simulink model "Our_PID_Plain"  (Simulink 8.9)
settings: Solver=VariableStepAuto  StartTime=0.0  StopTime=3000  RelTol=1e-3
settings Model: Creator=maurice waked  LastModifiedBy=maurice waked
settings DataIOCC: LimitDataPoints=off  SaveFormat=Dataset  SignalLoggingSaveFormat=Dataset  ReturnWorkspaceOutputs=on
settings OptimizationCC: LifeSpan=auto
settings DebuggingCC: UnderspecifiedInitializationDetection=Simplified  MergeDetectMultiDrivingBlocksExec=error  FcnCallInpInsideContextMsg=error  StateNameClashWarn=none  SFUnexpectedBacktrackingDiag=error  SFNoUnconditionalDefaultTransitionDiag=error  SFExecutionAtInitializationDiag=warning
settings HardwareCC: ProdBitPerPointer=64  ProdBitPerSizeT=64  ProdBitPerPtrDiffT=64  ProdLargestAtomicFloat=Float  ProdIntDivRoundTo=Zero  ProdEndianess=LittleEndian  ProdWordSize=64  ProdHWDeviceType=Intel->x86-64 (Windows64)
settings ModelReferenceCC: PropagateSignalLabelsOutOfModel=on
settings SFSimCC: SimUseLocalCustomCode=on
settings RTWCC: RTWUseLocalCustomCode=on
settings GRTTargetCC: TargetLangStandard=C99 (ISO)  CombineOutputUpdateFcns=on  GRTInterface=off
settings ConfigComp: CovMetricSettings=dwe  CovHtmlReporting=off  CovSaveCumulativeToWorkspaceVar=off  CovSaveSingleToWorkspaceVar=off  CovExternalEMLEnable=on

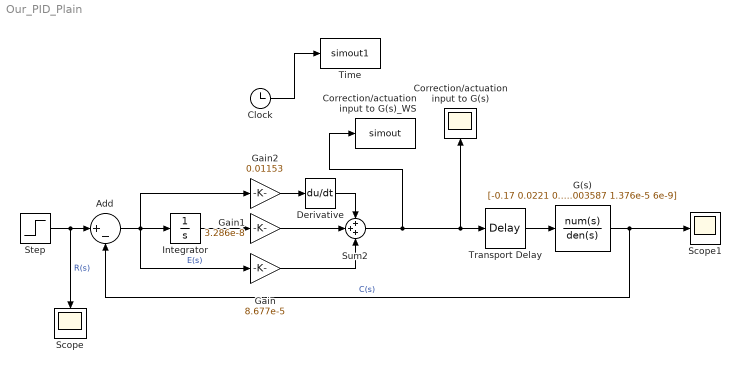
== system Our_PID_Plain ==
  Add : Sum  Inputs=|+-
  Clock : Clock
  Correction/actuation input to G(s) : Scope
  Correction/actuation input to G(s)_WS : ToWorkspace  VariableName=simout  SampleTime=-1
  Derivative : Derivative
  G(s) : TransferFcn  Numerator=[-0.17 0.0221 0.00068]  Denominator=[1 0.1345 0.003587 1.376e-5 6e-9]
  Gain : Gain  Gain=8.677e-5
  Gain1 : Gain  Gain=3.286e-8
  Gain2 : Gain  Gain=0.01153
  Integrator : Integrator
  Scope : Scope
  Scope1 : Scope
  Step : Step  Time=0  SampleTime=0
  Sum2 : Sum  Inputs=+++
  Time : ToWorkspace  VariableName=simout1  SampleTime=-1
  Transport Delay : TransportDelay  DelayTime=8.5
  wires:
  G(s)/1 -> Scope1/1, Add/2  "C(s)"
  Step/1 -> Add/1, Scope/1  "R(s)"
  Add/1 -> Gain2/1, Gain/1, Integrator/1  "E(s)"
  Gain1/1 -> Sum2/2
  Derivative/1 -> Sum2/1
  Gain/1 -> Sum2/3
  Integrator/1 -> Gain1/1
  Gain2/1 -> Derivative/1
  Sum2/1 -> Correction/actuation input to G(s)_WS/1, Transport Delay/1, Correction/actuation input to G(s)/1
  Clock/1 -> Time/1
  Transport Delay/1 -> G(s)/1
